simulink model "sampleModel1842"  (R2023a)
settings: Solver=VariableStepAuto  StartTime=0.0  StopTime=10.0  RelTol=1e-3
libraries: hdlsllib x3, simulink x1
settings Model: Creator=user1  LastModifiedBy=user1

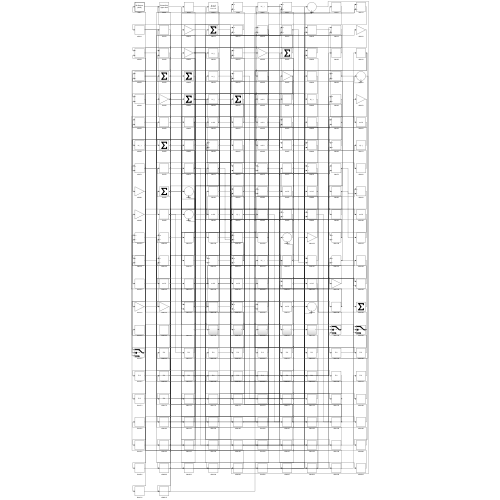
[thumbnail: Simulink's stored preview of the top-level diagram]
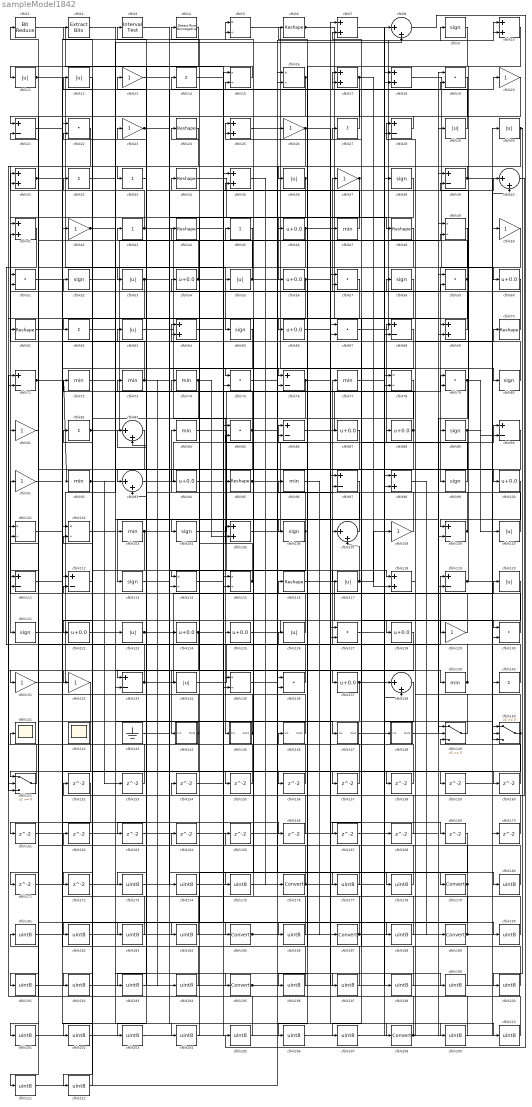
== system sampleModel1842 ==
  cfblk1 : hdlsllib/Logic and Bit Operations/Bit Reduce  mode=AND
  cfblk{7,10,17..18,25,31,35,41,64,69,98,105,118} (13 alike) : Sum
  cfblk{46,54,56,60,66,87..88,94,100,122,124..125,128,137} (14 alike) : Bias  Bias=0.0  SaturateOnIntegerOverflow=off
  cfblk{5,15..16,49,78,101..102,114..115,135} (10 alike) : Product  Inputs=*/  RndMeth=Zero  SaturateOnIntegerOverflow=on
  cfblk{47,72..74,77,84,92,96,103,139} (10 alike) : MinMax
  cfblk{9,38,52,58,65,80,89,99,104,106,113,121} (12 alike) : Signum
  cfblk{8,40,83,93,107,138} (6 alike) : Sum  Inputs=|++
  cfblk{13,20,23,26,37,42,50,81,91,108,129,131..132} (13 alike) : Gain
  cfblk{21,28,39,68,71,76,86,90,97,109,111..112,119,133} (14 alike) : Sum  Inputs=+-
  cfblk{11..12,29..30,36,53,55,63,110,117,120,123,126,134} (14 alike) : Abs  SaturateOnIntegerOverflow=off
  cfblk{6,24,34,44,48,61,70,95,116} (9 alike) : Reshape
  cfblk{19,22,51,57,59,67,75,79,85,127,130,136} (12 alike) : DotProduct  OutDataTypeStr=Inherit: Inherit via internal rule
  cfblk{14,27,32..33,43,45,62,82,140} (9 alike) : Sum  Inputs=+
  cfblk141 : Scope
  cfblk142 : Scope
      settings: Floating=on
  cfblk143 : Ground
  cfblk144 : Subsystem
      settings: LibrarySourceBlock=|
      | hdlsllib/Ports &
      | Subsystems/Subsystem
  cfblk145 : Subsystem
      settings: LibrarySourceBlock=|
      | hdlsllib/Ports &
      | Subsystems/Subsystem
  cfblk146 : Subsystem
      settings: LibrarySourceBlock=|
      | hdlsllib/Ports &
      | Subsystems/Subsystem
  cfblk147 : Subsystem
      settings: LibrarySourceBlock=|
      | hdlsllib/Ports &
      | Subsystems/Subsystem
  cfblk148 : Subsystem
      settings: LibrarySourceBlock=|
      | hdlsllib/Ports &
      | Subsystems/Subsystem
  cfblk149 : Switch  SaturateOnIntegerOverflow=off  InputSameDT=off
  cfblk150 : Switch  SaturateOnIntegerOverflow=off  InputSameDT=off
  cfblk151 : Switch  SaturateOnIntegerOverflow=off  InputSameDT=off
  cfblk{152..172} (21 alike) : Delay  SampleTime=1
  cfblk{173..175,177..178,180..184,186,188,190..194,196..207,209..212} (33 alike) : DataTypeConversion  OutDataTypeStr=uint8  SaturateOnIntegerOverflow=off  RndMeth=Floor
  cfblk{176,179,185,187,189,195,208} (7 alike) : DataTypeConversion  SaturateOnIntegerOverflow=off  RndMeth=Floor
  cfblk2 : simulink/Logic and Bit Operations/Extract Bits  bitsToExtract=Upper half  numBits=8  bitIdxRange=[0 7]  outScalingMode=Preserve fixed-point scaling
      settings: LibrarySourceBlock=|
      | hdlsllib/Logic and Bit
      | Operations/Extract Bits
  cfblk3 : hdlsllib/Logic and Bit Operations/Interval Test  IntervalClosedRight=on  uplimit=0.5  IntervalClosedLeft=on  lowlimit=-0.5  OutDataTypeStr=boolean
  cfblk4 : hdlsllib/Logic and Bit Operations/Detect Rise Nonnegative  vinit=0  OutDataTypeStr=boolean
  wires:
  cfblk110/1 -> cfblk84/1
  cfblk18/1 -> cfblk60/1
  cfblk63/1 -> cfblk75/1
  cfblk57/1 -> cfblk121/1
  cfblk60/1 -> cfblk25/1
  cfblk54/1 -> cfblk2/1, cfblk159/1
  cfblk41/1 -> cfblk119/1
  cfblk38/1 -> cfblk114/1
  cfblk68/1 -> cfblk104/1
  cfblk129/1 -> cfblk24/1
  cfblk15/1 -> cfblk11/1
  cfblk5/1 -> cfblk80/1
  cfblk48/1 -> cfblk65/1
  cfblk67/1 -> cfblk9/1
  cfblk13/1 -> cfblk185/1
  cfblk45/1 -> cfblk131/1
  cfblk43/1 -> cfblk145/1(In1), cfblk95/1, cfblk21/2, cfblk49/2
  cfblk126/1 -> cfblk91/1
  cfblk105/1 -> cfblk90/1
  cfblk71/1 -> cfblk92/1, cfblk70/1
  cfblk145/1(Out1) -> cfblk82/1, cfblk74/1
  cfblk97/1 -> cfblk113/1
  cfblk133/1 -> cfblk77/1, cfblk51/2
  cfblk84/1 -> cfblk118/1
  cfblk42/1 -> cfblk8/2, cfblk186/1
  cfblk127/1 -> cfblk179/1
  cfblk49/1 -> cfblk99/1
  cfblk107/1 -> cfblk4/1
  cfblk122/1 -> cfblk123/1
  cfblk6/1 -> cfblk148/1(In1), cfblk10/2
  cfblk11/1 -> cfblk55/1, cfblk130/2
  cfblk82/1 -> cfblk45/1, cfblk94/1
  cfblk93/1 -> cfblk68/1
  cfblk65/1 -> cfblk114/2
  cfblk101/1 -> cfblk208/1
  cfblk108/1 -> cfblk23/1
  cfblk29/1 -> cfblk5/1
  cfblk99/1 -> cfblk27/1
  cfblk123/1 -> cfblk116/1, cfblk130/1
  cfblk124/1 -> cfblk144/1(In1), cfblk17/2, cfblk120/1
  cfblk46/1 -> cfblk53/1, cfblk169/1
  cfblk81/1 -> cfblk111/1
  cfblk31/1 -> cfblk67/2, cfblk20/1
  cfblk12/1 -> cfblk62/1
  cfblk90/1 -> cfblk125/1
  cfblk149/1 -> cfblk73/1
  cfblk100/1 -> cfblk109/1
  cfblk102/1 -> cfblk195/1
  cfblk34/1 -> cfblk56/1
  cfblk70/1 -> cfblk37/1
  cfblk140/1 -> cfblk15/2
  cfblk85/1 -> cfblk12/1, cfblk135/2, cfblk177/1
  cfblk146/1(Out1) -> cfblk63/1
  cfblk23/1 -> cfblk109/2, cfblk178/1, cfblk199/1
  cfblk10/1 -> cfblk89/1
  cfblk24/1 -> cfblk81/1
  cfblk72/1 -> cfblk106/1
  cfblk62/1 -> cfblk139/1
  cfblk61/1 -> cfblk76/1
  cfblk147/1(Out1) -> cfblk38/1
  cfblk39/1 -> cfblk140/1, cfblk33/1
  cfblk95/1 -> cfblk79/1, cfblk97/2
  cfblk80/1 -> cfblk28/1
  cfblk106/1 -> cfblk22/2, cfblk212/1
  cfblk125/1 -> cfblk128/1
  cfblk17/1 -> cfblk93/1, cfblk118/2
  cfblk86/1 -> cfblk8/1
  cfblk89/1 -> cfblk110/1, cfblk161/1
  cfblk27/1 -> cfblk14/1
  cfblk104/1 -> cfblk26/1
  cfblk14/1 -> cfblk69/1
  cfblk139/1 -> cfblk107/1, cfblk57/2
  cfblk136/1 -> cfblk72/1
  cfblk1/1 -> cfblk115/1
  cfblk143/1 -> cfblk19/2
  cfblk134/1 -> cfblk28/2
  cfblk16/1 -> cfblk103/1, cfblk66/1
  cfblk114/1 -> cfblk40/1
  cfblk79/1 -> cfblk149/2, cfblk90/2
  cfblk109/1 -> cfblk6/1, cfblk64/2
  cfblk25/1 -> cfblk16/1
  cfblk92/1 -> cfblk79/2, cfblk153/1
  cfblk76/1 -> cfblk87/1, cfblk203/1
  cfblk131/1 -> cfblk17/1
  cfblk150/1 -> cfblk126/1, cfblk183/1
  cfblk137/1 -> cfblk150/3, cfblk155/1
  cfblk119/1 -> cfblk40/2, cfblk39/2
  cfblk37/1 -> cfblk41/1, cfblk132/1
  cfblk73/1 -> cfblk41/2, cfblk194/1, cfblk197/1
  cfblk148/1(Out1) -> cfblk69/2
  cfblk44/1 -> cfblk137/1
  cfblk74/1 -> cfblk122/1, cfblk105/2
  cfblk22/1 -> cfblk71/2
  cfblk19/1 -> cfblk61/1
  cfblk47/1 -> cfblk3/1
  cfblk58/1 -> cfblk151/1
  cfblk128/1 -> cfblk151/2
  cfblk96/1 -> cfblk187/1
  cfblk144/1(Out1) -> cfblk31/1, cfblk172/1
  cfblk36/1 -> cfblk86/2, cfblk193/1
  cfblk35/1 -> cfblk176/1
  cfblk30/1 -> cfblk76/2, cfblk196/1, cfblk200/1
  cfblk88/1 -> cfblk134/1, cfblk64/1
  cfblk28/1 -> cfblk21/1
  cfblk118/1 -> cfblk58/1
  cfblk87/1 -> cfblk135/1
  cfblk55/1 -> cfblk44/1, cfblk10/1
  cfblk52/1 -> cfblk147/1(In1)
  cfblk3/1 -> cfblk48/1
  cfblk91/1 -> cfblk42/1
  cfblk116/1 -> cfblk150/2
  cfblk2/1 -> cfblk100/1
  cfblk151/1 -> cfblk141/1
  cfblk103/1 -> cfblk43/1, cfblk117/1, cfblk202/1
  cfblk121/1 -> cfblk5/2
  cfblk56/1 -> cfblk129/1, cfblk175/1
  cfblk33/1 -> cfblk133/1
  cfblk53/1 -> cfblk151/3, cfblk59/2, cfblk133/2
  cfblk69/1 -> cfblk51/1
  cfblk59/1 -> cfblk31/2, cfblk167/1
  cfblk98/1 -> cfblk189/1
  cfblk66/1 -> cfblk47/1
  cfblk117/1 -> cfblk107/2, cfblk108/1
  cfblk20/1 -> cfblk36/1
  cfblk115/1 -> cfblk34/1, cfblk105/1
  cfblk130/1 -> cfblk86/1
  cfblk26/1 -> cfblk136/2, cfblk210/1
  cfblk153/1 -> cfblk71/1
  cfblk40/1 -> cfblk154/1
  cfblk154/1 -> cfblk115/2
  cfblk155/1 -> cfblk1/1
  cfblk9/1 -> cfblk156/1
  cfblk156/1 -> cfblk15/1
  cfblk135/1 -> cfblk157/1
  cfblk157/1 -> cfblk25/2
  cfblk75/1 -> cfblk158/1
  cfblk158/1 -> cfblk93/2
  cfblk159/1 -> cfblk150/1
  cfblk51/1 -> cfblk160/1
  cfblk160/1 -> cfblk149/3
  cfblk161/1 -> cfblk39/1
  cfblk162/1 -> cfblk59/1
  cfblk4/1 -> cfblk163/1
  cfblk164/1 -> cfblk85/1
  cfblk165/1 -> cfblk119/2
  cfblk111/1 -> cfblk166/1
  cfblk166/1 -> cfblk22/1
  cfblk167/1 -> cfblk68/2
  cfblk77/1 -> cfblk168/1
  cfblk168/1 -> cfblk18/1
  cfblk170/1 -> cfblk149/1
  cfblk132/1 -> cfblk171/1
  cfblk171/1 -> cfblk16/2
  cfblk172/1 -> cfblk124/1
  cfblk78/1 -> cfblk173/1
  cfblk173/1 -> cfblk18/2
  cfblk163/1 -> cfblk174/1
  cfblk174/1 -> cfblk78/1
  cfblk175/1 -> cfblk78/2
  cfblk176/1 -> cfblk57/1, cfblk111/2
  cfblk177/1 -> cfblk35/1
  cfblk178/1 -> cfblk35/2
  cfblk179/1 -> cfblk52/1, cfblk191/1
  cfblk94/1 -> cfblk180/1
  cfblk180/1 -> cfblk127/1
  cfblk181/1 -> cfblk127/2
  cfblk112/1 -> cfblk182/1
  cfblk182/1 -> cfblk46/1
  cfblk183/1 -> cfblk112/1
  cfblk169/1 -> cfblk184/1
  cfblk184/1 -> cfblk112/2
  cfblk185/1 -> cfblk30/1, cfblk67/1
  cfblk186/1 -> cfblk13/1
  cfblk187/1 -> cfblk162/1, cfblk85/2, cfblk49/1
  cfblk64/1 -> cfblk188/1
  cfblk188/1 -> cfblk96/1
  cfblk189/1 -> cfblk165/1, cfblk164/1
  cfblk21/1 -> cfblk190/1
  cfblk190/1 -> cfblk98/1
  cfblk191/1 -> cfblk98/2
  cfblk83/1 -> cfblk192/1
  cfblk192/1 -> cfblk19/1
  cfblk193/1 -> cfblk83/1
  cfblk194/1 -> cfblk83/2
  cfblk195/1 -> cfblk170/1, cfblk97/1
  cfblk196/1 -> cfblk102/1
  cfblk197/1 -> cfblk102/2
  cfblk7/1 -> cfblk198/1
  cfblk198/1 -> cfblk146/1(In1)
  cfblk199/1 -> cfblk7/1
  cfblk200/1 -> cfblk7/2
  cfblk138/1 -> cfblk201/1
  cfblk201/1 -> cfblk75/2
  cfblk202/1 -> cfblk138/1
  cfblk203/1 -> cfblk138/2
  cfblk32/1 -> cfblk204/1
  cfblk204/1 -> cfblk54/1
  cfblk8/1 -> cfblk205/1
  cfblk205/1 -> cfblk32/1
  cfblk50/1 -> cfblk206/1
  cfblk206/1 -> cfblk29/1
  cfblk120/1 -> cfblk207/1
  cfblk207/1 -> cfblk50/1
  cfblk208/1 -> cfblk181/1, cfblk88/1
  cfblk113/1 -> cfblk209/1
  cfblk209/1 -> cfblk101/1
  cfblk210/1 -> cfblk101/2
  cfblk152/1 -> cfblk211/1
  cfblk211/1 -> cfblk136/1
  cfblk212/1 -> cfblk152/1

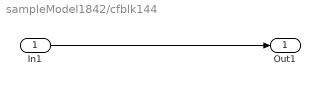
== system sampleModel1842/cfblk144 ==
  In1 : Inport
  Out1 : Outport
  wires:
  In1/1 -> Out1/1

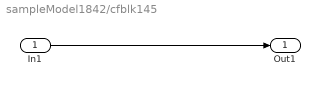
== system sampleModel1842/cfblk145 ==
  In1 : Inport
  Out1 : Outport
  wires:
  In1/1 -> Out1/1

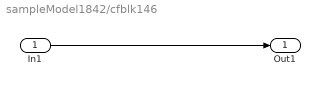
== system sampleModel1842/cfblk146 ==
  In1 : Inport
  Out1 : Outport
  wires:
  In1/1 -> Out1/1

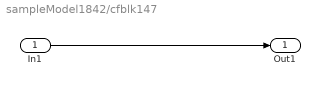
== system sampleModel1842/cfblk147 ==
  In1 : Inport
  Out1 : Outport
  wires:
  In1/1 -> Out1/1

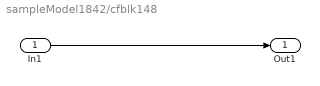
== system sampleModel1842/cfblk148 ==
  In1 : Inport
  Out1 : Outport
  wires:
  In1/1 -> Out1/1
